simulink model "TrajectoryFollowVehicleWith14DoF"  (R2024a)
settings: Solver=VariableStepAuto  StartTime=0  StopTime=14  FixedStep=timeStep  RelTol=1e-3
PreLoadFcn:
  | useDynamicsStanley = false; %Simulink model to move according to the scenario trajectory.
  | vehicleVariant = "3DOF";
PostLoadFcn:
  | load(fullfile(matlabroot,'toolbox','driving','drivingdata','rrScenarioSimTypes.mat'));
  | helperSLTrajectoryFollowerWithRRScenarioSetup();
  | heightMap = "flat";
  | if isfile("pathFollowingUtil/gridMap_groundHeight_RT.mat")
  |     load("gridMap_groundHeight_RT.mat");
  | end
  | % if exist("z_2DTable", "var") && exist("xBreakPts", "var") && exist("yBreakPts", "var")
  | %     hegihtMap = "2DMap";
  | % end
  | % if isfile("CRG/crgRoad.crg")
  | %     crgData = crg_read('CRG/crgRoad.crg');
  | % end
InitFcn:
  | if ~exist("useLongitudinalEV", "var")
  |     useLongitudinalEV = false;
  | end
StartFcn:
  | % set_param(bdroot, 'Profile', 'on');
StopFcn:
  | % set_param(bdroot, 'Profile', 'off');
  | % slprofreport(bdroot, 'report14DoF.html');
undefined symbols (not defined in the file or in its folder): ActorRuntime, Camera, control_timeStep, Defined, DiscIntNeverNeededParam, dz, Ego, egoInitialPose, egoInitialPoseCG, egoInitialPoseRear, InitVehicle, kmph2mps, Lane, lr, m, magnitude, max_dc, n, numReferencePose, pitch, roll, RRtimeStep, SceneData, SRE, steerGear, tau, tau2, timeStep, User, VehicleData, WheelPoses, X, xBreakPts, Y, yaw, yBreakPts, Z, z_2DTable
libraries: sm_lib x108, nesl_utility x62, sm_vehicle_utilities_lib x30, simulink_extras x12, roadrunnerscenario x6, simulink x4, drivingvehiclecontroller x4, autolibshared x2, mpcadaslib x2, autolibutils x1, METI_Lib_vehicle_model x1
(part 2 of 6)

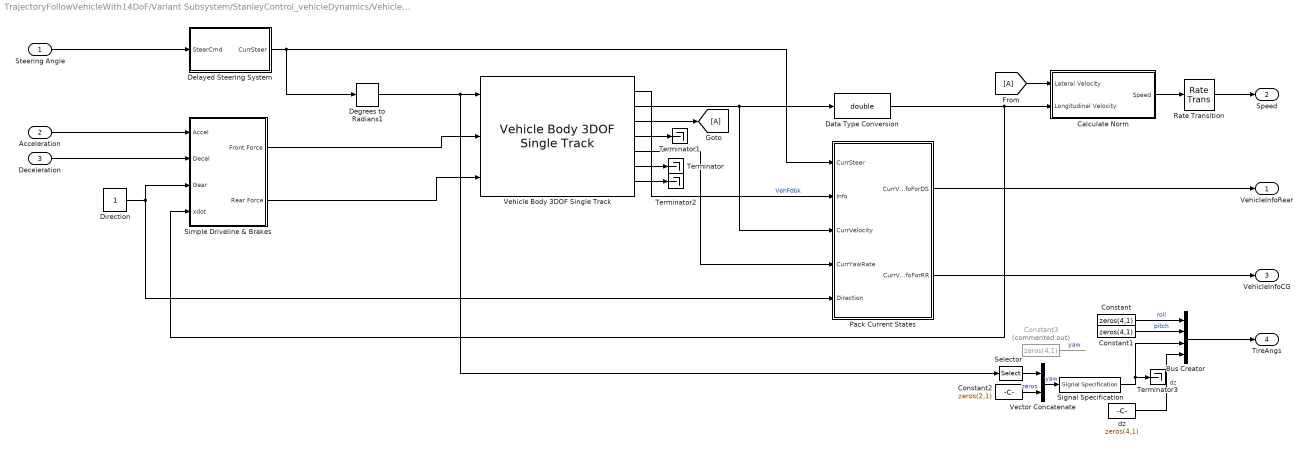
== system TrajectoryFollowVehicleWith14DoF/Variant Subsystem/StanleyControl_vehicleDynamics/Vehicle Dynamics1/Vehicle Dynamics 3DOF ==
  Steering Angle : Inport
  Acceleration : Inport  Port=2
  Deceleration : Inport  Port=3
  Bus Creator : BusCreator  Inputs=roll,pitch,yaw,dz
  Calculate Norm : Subsystem
  Constant : Constant  Value=zeros(4,1)
  Constant1 : Constant  Value=zeros(4,1)
  Constant2 : Constant  Value=zeros(2,1)
  Constant3 : Constant  Commented=on  Value=zeros(4,1)
  Data Type Conversion : DataTypeConversion  OutDataTypeStr=double  SaturateOnIntegerOverflow=off  RndMeth=Floor
  Degrees to Radians1 : simulink_extras/Transformations/Degrees to Radians
  Delayed Steering System : Subsystem
  Direction : Constant
  From : From
  Goto : Goto
  Pack Current States : Subsystem
  Rate Transition : RateTransition
  Selector : Selector  InputPortWidth=1  IndexOptions=Index vector (dialog)  Indices=[1; 1]  OutputSizes=1
  Signal Specification : SignalSpecification  Unit=rad  Dimensions=[4,1]
  Simple Driveline & Brakes : Subsystem
  Terminator{,1..3} (4 alike) : Terminator
  Vector Concatenate : Concatenate  Mode=Multidimensional array
  Vehicle Body 3DOF Single Track : autolibshared/Vehicle Body 3DOF Single Track  trackMode=Single (bicycle)  inputMode=External longitudinal forces  frontSteerMode=on  rearSteerMode=off  windMode=off  muMode=off  extFMode=off  extMMode=off  htchFMode=off  htchMMode=off  extXo=off  extpsio=off  extxdoto=off  extro=off  extYo=off  extTamb=off  extydoto=off  aMode=2  NF=2  NR=2  m=m  a=lf  b=lr  h=0.35  dh=1  hh=0.2  X_o=egoInitialPoseCG.CurrPose(1)  xdot_o=egoInitialPoseCG.CurrVelocity  CalphaMode=off  sigmaMode=off  d=0  hl=0  w=[1.4,1.4]  Cy_f=Cf  Cy_r=Cr  sigma_f=.1  sigma_r=.1  alpha_f_brk=[-.1 .1]  Cy_f_data=[-9e3 9e3]  alpha_r_brk=[-.1 .1]  Cy_r_data=[-9e3 9e3]  Y_o=egoInitialPoseCG.CurrPose(2)  ydot_o=0  Izz=Iz  psi_o=deg2rad(egoInitialPoseCG.CurrPose(3))  r_o=deg2rad(egoInitialPoseCG.CurrYawRate)  Af=0  Cd=.3  Cl=.1  Cpm=.1  beta_w=[0:0.01:0.3]  Cs=[0:0.03:0.9]  Cym=[0:0.01:0.3]  Pabs=101325  Tair=273  g=9.81  mu=1  xdot_tol=.01  Fznom=5000  Fxtire_sat=7e4  Fytire_sat=7e4  longOff=0  latOff=0  vertOff=0  wrapAng=off
  dz : Constant  Value=zeros(4,1)
  VehicleInfoRear : Outport
  Speed : Outport  Port=2
  VehicleInfoCG : Outport  Port=3
  TireAngs : Outport  Port=4
  wires:
  Steering Angle/1 -> Delayed Steering System/1(SteerCmd)
  Acceleration/1 -> Simple Driveline & Brakes/1(Accel)
  Calculate Norm/1(Speed) -> Rate Transition/1
  Direction/1 -> Pack Current States/5(Direction), Simple Driveline & Brakes/3(Gear)
  Simple Driveline & Brakes/1(Front Force) -> Vehicle Body 3DOF Single Track/2
  Vehicle Body 3DOF Single Track/5 -> Pack Current States/4(CurrYawRate)
  Vehicle Body 3DOF Single Track/4 -> Terminator1/1
  Degrees to Radians1/1 -> Selector/1, Vehicle Body 3DOF Single Track/1
  Delayed Steering System/1(CurrSteer) -> Degrees to Radians1/1, Pack Current States/1(CurrSteer)
  Pack Current States/1(CurrVehicleInfoForDS) -> VehicleInfoRear/1
  Rate Transition/1 -> Speed/1
  Simple Driveline & Brakes/2(Rear Force) -> Vehicle Body 3DOF Single Track/3
  From/1 -> Calculate Norm/1(Lateral Velocity)
  Vehicle Body 3DOF Single Track/2 -> Data Type Conversion/1, Pack Current States/3(CurrVelocity)
  Vehicle Body 3DOF Single Track/6 -> Terminator/1
  Deceleration/1 -> Simple Driveline & Brakes/2(Decel)
  Vehicle Body 3DOF Single Track/7 -> Terminator2/1
  Vehicle Body 3DOF Single Track/3 -> Goto/1
  Data Type Conversion/1 -> Calculate Norm/2(Longitudinal Velocity), Simple Driveline & Brakes/4(xdot)
  Vehicle Body 3DOF Single Track/1 -> Pack Current States/2(Info)  "VehFdbk"
  Pack Current States/2(CurrVehicleInfoForRR) -> VehicleInfoCG/1
  Constant/1 -> Bus Creator/1  "roll"
  Constant1/1 -> Bus Creator/2  "pitch"
  Bus Creator/1 -> TireAngs/1
  Vector Concatenate/1 -> Signal Specification/1  "yaw"
  Constant2/1 -> Vector Concatenate/2  "zeros"
  dz/1 -> Bus Creator/4  "dz"
  Constant3/1 -> ?  "yaw"
  Selector/1 -> Vector Concatenate/1
  Signal Specification/1 -> Bus Creator/3, Terminator3/1

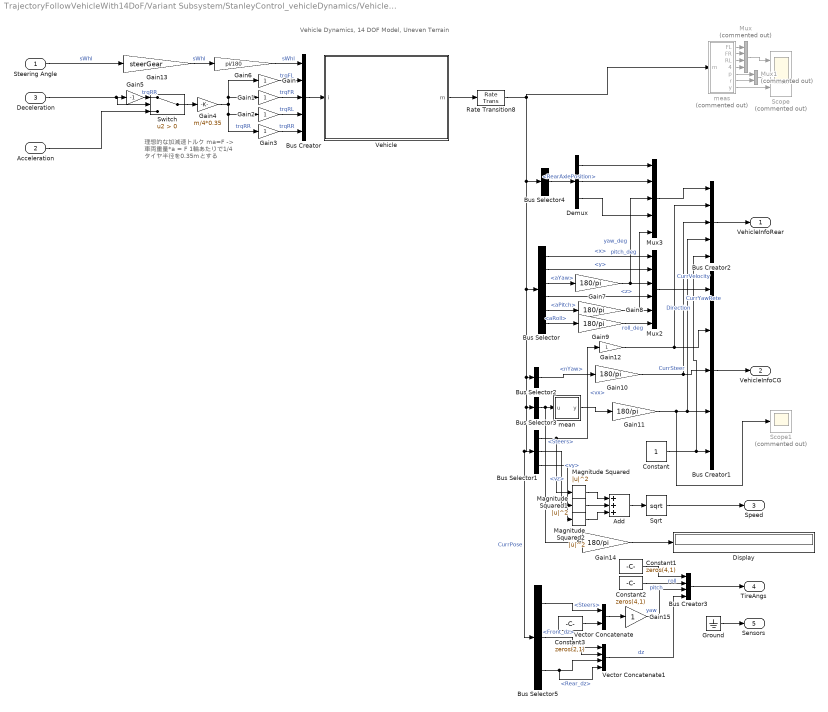
== system TrajectoryFollowVehicleWith14DoF/Variant Subsystem/StanleyControl_vehicleDynamics/Vehicle Dynamics1/Vehicle Dynamics Multibody ==
  note: 理想的な加減速トルク
      | ma=F -> 車両重量*a = F
      | 1輪あたりで1/4
      | タイヤ半径を0.35mとする
  note: Vehicle Dynamics, 14 DOF Model, Uneven Terrain
  Steering Angle : Inport
  Acceleration : Inport  Port=2
  Deceleration : Inport  Port=3
  Add : Sum  Inputs=+++
  Bus Creator : BusCreator  Inputs=5
  Bus Creator1 : BusCreator  Inputs=5  OutDataTypeStr=Bus: BusFullVehicleInfo  NonVirtualBus=on
      settings: InheritFromInputs=off
  Bus Creator2 : BusCreator  Inputs=5  OutDataTypeStr=Bus: BusVehicleInfo  NonVirtualBus=on
      settings: InheritFromInputs=off
  Bus Creator3 : BusCreator  Inputs=4
  Bus Selector : BusSelector  OutputSignals=Body.x,Body.y,Body.aYaw,Body.z,Body.aPitch,Body.aRoll
  Bus Selector1 : BusSelector  OutputSignals=Body.vx,Body.vy,Body.vz
  Bus Selector2 : BusSelector  OutputSignals=Body.nYaw
  Bus Selector3 : BusSelector  OutputSignals=Steers
  Bus Selector4 : BusSelector  OutputSignals=RearAxlePosition
  Bus Selector5 : BusSelector  OutputSignals=Steers,Front_dz,Rear_dz
  Constant : Constant
  Constant1 : Constant  Value=zeros(4,1)
  Constant2 : Constant  Value=zeros(4,1)
  Constant3 : Constant  Value=zeros(2,1)
  Demux : Demux  Outputs=3
  Display : Display
  Gain{,1..3,12,15} (6 alike) : Gain
  Gain{7..11,14} (6 alike) : Gain  Gain=180/pi
  Gain13 : Gain  Gain=steerGear
  Gain4 : Gain  Gain=m/4*0.35
  Gain5 : Gain  Gain=-1
  Gain6 : Gain  Gain=pi/180
  Ground : Ground
  Magnitude Squared : Math  Operator=magnitude^2
  Magnitude Squared1 : Math  Operator=magnitude^2
  Magnitude Squared2 : Math  Operator=magnitude^2
  Mux : Mux  Commented=on
  Mux1 : Mux  Commented=on  Inputs=2
  Mux2 : Mux  Inputs=6
  Mux3 : Mux  Inputs=5
  Rate Transition8 : RateTransition  OutPortSampleTime=timeStep
  Scope : Scope  Commented=on  NumInputPorts=3
  Scope1 : Scope  Commented=on
  Sqrt : Sqrt  OutputSignalType=real
  Switch : Switch  Criteria=u2 > Threshold  SaturateOnIntegerOverflow=off  InputSameDT=off
  Vector Concatenate : Concatenate
  Vector Concatenate1 : Concatenate  NumInputs=4
  Vehicle : Subsystem  mask(Vehicle and Scene){vehdata=VehicleData, initveh=InitVehicle}
      mask prompts: vehdata "Vehicle Data (structure)"; initveh "Initial Position, Velocity (structure)"
      mask help: Models a vehicle with a configurable scene. Vehicle parameters are defined within a single data structure. A separate data structure defines the initial position, orientation, and speed of the vehicle and the wheels.
      settings: AttributesFormatString=%<popup_scene>
      mask Display:
      | image(['sm_vehicle_2axle_heave_roll_vehicle_grid_ray_trace.png']);
      | % Notes for mask images
      | % Screenshot taken MechExp 931x463, one pane 619x314
      | % Trim to 434 x 272, resize to 500x330
  mean : MATLAB Function  TreatAsAtomicUnit=on
  meas : Subsystem  Commented=on
  VehicleInfoRear : Outport
  VehicleInfoCG : Outport  Port=2
  Speed : Outport  Port=3
  TireAngs : Outport  Port=4
  Sensors : Outport  Port=5
  wires:
  Demux/3 -> Mux3/4
  Magnitude Squared2/1 -> Add/3
  Gain11/1 -> Scope1/1, Bus Creator1/4, Bus Creator2/4  "CurrSteer"
  Demux/1 -> Mux3/1
  Bus Creator1/1 -> VehicleInfoCG/1
  Bus Selector1/1 -> Gain12/1, Magnitude Squared/1  "<vx>"
  Bus Creator2/1 -> VehicleInfoRear/1
  Mux2/1 -> Bus Creator1/1
  Bus Selector/4 -> Mux2/4  "<z>"
  Gain13/1 -> Gain6/1  "sWhl"
  Gain6/1 -> Bus Creator/1  "sWhl"
  Sqrt/1 -> Speed/1
  Bus Selector1/2 -> Magnitude Squared1/1  "<vy>"
  Bus Selector3/1 -> Gain14/1, mean/1(u)  "<Steers>"
  Bus Selector/5 -> Gain8/1  "<aPitch>"
  Gain12/1 -> Bus Creator1/2, Bus Creator2/2  "CurrVelocity"
  Bus Selector2/1 -> Gain10/1  "<nYaw>"
  Gain10/1 -> Bus Creator2/3, Bus Creator1/3  "CurrYawRete"
  Bus Selector/1 -> Mux2/1  "<x>"
  Constant/1 -> Bus Creator2/5, Bus Creator1/5  "Direction"
  Mux3/1 -> Bus Creator2/1
  Bus Selector/2 -> Mux2/2  "<y>"
  Magnitude Squared/1 -> Add/1
  Magnitude Squared1/1 -> Add/2
  Gain7/1 -> Mux3/3, Mux2/3  "yaw_deg"
  Acceleration/1 -> Switch/3
  Mux/1 -> Scope/1
  meas/3(RL) -> Mux/3
  Demux/2 -> Mux3/2
  Bus Selector1/3 -> Magnitude Squared2/1  "<vz>"
  Vehicle/1(m) -> Rate Transition8/1
  Gain3/1 -> Bus Creator/5  "trqRR"
  Bus Selector/3 -> Gain7/1  "<aYaw>"
  Switch/1 -> Gain4/1
  Gain4/1 -> Gain1/1, Gain/1, Gain2/1, Gain3/1  "trqRR"
  Add/1 -> Sqrt/1
  Gain5/1 -> Switch/1  "trqRR"
  Gain/1 -> Bus Creator/2  "trqFL"
  mean/1(y) -> Gain11/1
  Bus Creator/1 -> Vehicle/1(i)
  meas/2(FR) -> Mux/2
  meas/1(FL) -> Mux/1
  Gain1/1 -> Bus Creator/3  "trqFR"
  Gain9/1 -> Mux2/6  "roll_deg"
  meas/6(r) -> Mux1/2
  meas/7(y) -> Scope/3
  Steering Angle/1 -> Gain13/1  "sWhl"
  Deceleration/1 -> Switch/2, Gain5/1
  Mux1/1 -> Scope/2
  meas/4(RR) -> Mux/4
  Gain8/1 -> Mux3/5, Mux2/5  "pitch_deg"
  Bus Selector4/1 -> Demux/1  "<RearAxlePosition>"
  Gain2/1 -> Bus Creator/4  "trqRL"
  Bus Selector/6 -> Gain9/1  "<aRoll>"
  meas/5(p) -> Mux1/1
  Rate Transition8/1 -> meas/1(m), Bus Selector5/1, Bus Selector1/1, Bus Selector3/1, Bus Selector2/1, Bus Selector/1, Bus Selector4/1  "CurrPose"
  Gain14/1 -> Display/1
  Vector Concatenate/1 -> Gain15/1
  Constant1/1 -> Bus Creator3/1  "roll"
  Constant2/1 -> Bus Creator3/2  "pitch"
  Gain15/1 -> Bus Creator3/3  "yaw"
  Bus Creator3/1 -> TireAngs/1
  Vector Concatenate1/1 -> Bus Creator3/4  "dz"
  Ground/1 -> Sensors/1
  Constant3/1 -> Vector Concatenate/2
  Bus Selector5/1 -> Vector Concatenate/1  "<Steers>"
  Bus Selector5/2 -> Vector Concatenate1/2, Vector Concatenate1/1  "<Front_dz>"
  Bus Selector5/3 -> Vector Concatenate1/4, Vector Concatenate1/3  "<Rear_dz>"

== system TrajectoryFollowVehicleWith14DoF/Variant Subsystem/LongitudinalEV/VDBS_PTBS/Controllers/Powertrain Control Input ==
  OpCmds : Inport
  VehPlnt : Inport  Port=2
  Bus Selector1 : BusSelector  OutputSignals=Veh.xdot,Veh.MotSpd,Elec.BMS_Sensors
  Bus Selector2 : BusSelector  OutputSignals=Accel,Decel
  Rate Transition{,1..2,6} (4 alike) : RateTransition  Deterministic=off
  AccelPdl : Outport  VectorParamsAs1DForOutWhenUnconnected=off
  DecelPdl : Outport  Port=2  VectorParamsAs1DForOutWhenUnconnected=off
  VehSpdFdbk : Outport  Port=3  VectorParamsAs1DForOutWhenUnconnected=off
  MotSpd : Outport  Port=4  VectorParamsAs1DForOutWhenUnconnected=off
  BMS_Sensors : Outport  Port=5  OutDataTypeStr=Bus: Sensors  VectorParamsAs1DForOutWhenUnconnected=off
  wires:
  OpCmds/1 -> Bus Selector2/1
  VehPlnt/1 -> Bus Selector1/1
  Bus Selector2/1 -> Rate Transition/1  "<Accel>"
  Bus Selector2/2 -> Rate Transition1/1  "<Decel>"
  Bus Selector1/1 -> Rate Transition2/1  "<xdot>"
  Bus Selector1/2 -> Rate Transition6/1  "<MotSpd>"
  Rate Transition/1 -> AccelPdl/1
  Rate Transition1/1 -> DecelPdl/1
  Rate Transition2/1 -> VehSpdFdbk/1
  Rate Transition6/1 -> MotSpd/1
  Bus Selector1/3 -> BMS_Sensors/1  "<BMS_Sensors>"

== system TrajectoryFollowVehicleWith14DoF/Variant Subsystem/LongitudinalEV/VDBS_PTBS/Controllers/Powertrain Control Module (PCM) ==
  AccCmd : Inport
  DecCmd : Inport  Port=2
  VehSpdFdbk : Inport  Port=3
  MotSpd : Inport  Port=4
  BMS_Sensors : Inport  Port=5  OutDataTypeStr=Bus: Sensors
  Battery Management System (BMS) : ModelReference  ModelNameDialog=BMS_Software.slx  ModelReferenceVersion=8.0
  Enumerated Constant : simulink/Sources/Enumerated Constant  OutDataTypeStr=Enum: SRE  Value=SRE.Driving  SampleTime=inf
  Powertrain Control Module (PCM) : ModelReference  ModelNameDialog=EvPowertrainController.slx  ModelReferenceVersion=8.4
  MotTrqCmd : Outport
  BrakeCmd : Outport  Port=2
  BMS_Info : Outport  Port=3  OutDataTypeStr=Bus: BMS_Info
  BMS_Cmd : Outport  Port=4  OutDataTypeStr=Bus: BMS_Cmd
  wires:
  DecCmd/1 -> Powertrain Control Module (PCM)/2
  Powertrain Control Module (PCM)/1 -> MotTrqCmd/1
  [BMS_Info] -> Powertrain Control Module (PCM)/4
  MotSpd/1 -> Powertrain Control Module (PCM)/6
  VehSpdFdbk/1 -> Powertrain Control Module (PCM)/3
  AccCmd/1 -> Powertrain Control Module (PCM)/1
  Powertrain Control Module (PCM)/2 -> BrakeCmd/1
  Enumerated Constant/1 -> Battery Management System (BMS)/1
  Battery Management System (BMS)/1 -> [BMS_Info], BMS_Info/1
  Battery Management System (BMS)/2 -> [BMS_Cmd], BMS_Cmd/1
  BMS_Sensors/1 -> Powertrain Control Module (PCM)/7, Battery Management System (BMS)/2
  [BMS_Cmd] -> Powertrain Control Module (PCM)/5

== system TrajectoryFollowVehicleWith14DoF/Variant Subsystem/LongitudinalEV/VDBS_PTBS/Controllers/Powertrain Control Output ==
  MotTrqCmd : Inport
  BrkCmd : Inport  Port=2
  BMS_Info : Inport  Port=3  OutDataTypeStr=Bus: BMS_Info
  BMS_Cmd : Inport  Port=4  OutDataTypeStr=Bus: BMS_Cmd
  Bus Creator : BusCreator  Inputs=4
  PtCtrl : Outport  VectorParamsAs1DForOutWhenUnconnected=off
  wires:
  BrkCmd/1 -> Bus Creator/2  "BrkCmd"
  Bus Creator/1 -> PtCtrl/1  "PtCtrl"
  MotTrqCmd/1 -> Bus Creator/1  "MotTrqCmd"
  BMS_Info/1 -> Bus Creator/3  "BMS_Info"
  BMS_Cmd/1 -> Bus Creator/4  "BMS_Cmd"

== system TrajectoryFollowVehicleWith14DoF/Variant Subsystem/LongitudinalEV/VDBS_PTBS/Longitudinal Driver/Longitudinal Driver ==
  Vref : Inport
  Vfdbk : Inport  Port=2
  Bus Selector : BusSelector  OutputSignals=Veh.xdot
  Ground : Ground
  Longitudinal Driver Model : autolibshared/Longitudinal Driver  extAccelOvr=off  extDecelOvr=off  extAccelHld=off  extDecelHld=off  extAccelZero=off  extDecelZero=off  cntrlType=Predictive  shftType=Reverse, Neutral, Drive  velUnits=m/s  gearOut=off  Kp=1  Ki=1  Kff=0  Kg=0  VehVelVec=[0 100]  KffVec=[.1 .1]  KpVec=[10 10]  KiVec=[5 5]  KgVec=[0 0]  m=1645  Kpt=450*9.04/0.324  tau=0.12  L=4  aR=30.3/3875  bR=0.21290*4.44822/0.44704  cR=0.01278*4.44822/0.44704^2  g=9.81  vnom=1  Kaw=0  tauerr=0  tauPt=2  GearInit=0  tShift=.1  pdlVec=[0.1 0.4 0.5 0.9]  upShftTbl=[-1 12.9375 26.4375 39.9375 51.18749999999999 62.4375 72.84375 83.25;-1 16.3125 29.8125 43.3125 54.5624 65.8125 76.78125 87.75;-1 19.6875 33.1875 46.68749999999999 57.9375 69.1875 80.71875 92.25;-1 33 52.5 77.25 100.5 138.75 161.875 185]  dwnShftTbl=[1 9.5625 23.0625 36.5625 47.8125 59.0625 68.90625 78.75;1 12.9375 26.4375 39.9375 51.18749999999999 62.4375 72.84375 83.25;1 16.3125 29.8125 43.3125 54.562499 65.8125 76.78125 87.75;1 19.6875 33.1875 46.68749999999999 57.9375 69.1875 80.71875 92.25]  tClutch=.5  tRev=.5  tPark=120  aMode=1  UpGearVec="[0  1  2  3  4  5  6  7]"  DownGearVec="[1  2  3  4  5  6  7  8]"
  Terminator1 : Terminator
  OpCmds : Outport  VectorParamsAs1DForOutWhenUnconnected=off
  tag scope: Accel_VDBS=global
  wires:
  Bus Selector/1 -> Longitudinal Driver Model/2  "<xdot>"
  Vref/1 -> Longitudinal Driver Model/1  "xdotref"
  Vfdbk/1 -> Bus Selector/1
  Longitudinal Driver Model/2 -> [Accel_VDBS]  "Acc"
  Longitudinal Driver Model/3 -> Terminator1/1  "Dec"
  Ground/1 -> Longitudinal Driver Model/3
  Longitudinal Driver Model/1 -> OpCmds/1  "Info"

== system TrajectoryFollowVehicleWith14DoF/Variant Subsystem/LongitudinalEV/VDBS_PTBS/Longitudinal Driver/Open Loop ==
  note: This subsystem is provided to disable the driver subsystem and expose the driver interface.
      |
      | The interface can:
      | - be connected with dashboard UI blocks or 3rd party hardware
      | - provide application specific pre-programmed event or time based signals
      | - be driven by recorded operator signals for tuning, troubleshooting and model validation
  Bus Creator2 : BusCreator  Inputs=8
  Constant{1..4} (4 alike) : Constant  Value=0
  Ground{,1..3} (4 alike) : Ground
  OpCmds : Outport  VectorParamsAs1DForOutWhenUnconnected=off
  wires:
  Ground3/1 -> Bus Creator2/8  "ErrMin"
  Ground1/1 -> Bus Creator2/6  "ErrSqrSum"
  Bus Creator2/1 -> OpCmds/1  "Info"
  Ground2/1 -> Bus Creator2/7  "ErrMax"
  Constant1/1 -> Bus Creator2/1  "Accel"
  Constant3/1 -> Bus Creator2/3  "Gear"
  Constant2/1 -> Bus Creator2/2  "Decel"
  Ground/1 -> Bus Creator2/5  "Err"
  Constant4/1 -> Bus Creator2/4  "Clutch"

== system TrajectoryFollowVehicleWith14DoF/Variant Subsystem/LongitudinalEV/VDBS_PTBS/Passenger Car/Drivetrain Output ==
  VehSpd : Inport
  MotSpd : Inport  Port=2
  Bus Creator1 : BusCreator  Inputs=2
  VehFdbk : Outport  VectorParamsAs1DForOutWhenUnconnected=off
  wires:
  Bus Creator1/1 -> VehFdbk/1  "VehFdbk"
  VehSpd/1 -> Bus Creator1/1
  MotSpd/1 -> Bus Creator1/2  "MotSpd"

== system TrajectoryFollowVehicleWith14DoF/Variant Subsystem/LongitudinalEV/VDBS_PTBS/Passenger Car/Drivetrain Plant Input ==
  Ctrl : Inport
  ElecFdbk : Inport  Port=2
  Env : Inport  Port=3
  Bus Selector : BusSelector  OutputSignals=BrkCmd
  Bus Selector1 : BusSelector  OutputSignals=MotTrq
  Bus Selector3 : BusSelector  OutputSignals=Ground.Grade,Wind.wind_x
  First Order Hold : FirstOrderHold  ErrorTolerance=inf
  Rate Transition6 : RateTransition  Deterministic=off
  Rate Transition7 : RateTransition  Deterministic=off
  MotTrq : Outport  VectorParamsAs1DForOutWhenUnconnected=off
  BrkCmd : Outport  Port=2  VectorParamsAs1DForOutWhenUnconnected=off
  Grade : Outport  Port=3  VectorParamsAs1DForOutWhenUnconnected=off
  WindVel : Outport  Port=4  VectorParamsAs1DForOutWhenUnconnected=off
  wires:
  Ctrl/1 -> Bus Selector/1
  Bus Selector/1 -> First Order Hold/1  "<BrkCmd>"
  First Order Hold/1 -> BrkCmd/1  "BrkCmd"
  ElecFdbk/1 -> Bus Selector1/1
  Bus Selector1/1 -> MotTrq/1  "<MotTrq>"
  Env/1 -> Bus Selector3/1
  Rate Transition6/1 -> Grade/1  "Grade"
  Rate Transition7/1 -> WindVel/1  "WindVel"
  Bus Selector3/1 -> Rate Transition6/1  "<Grade>"
  Bus Selector3/2 -> Rate Transition7/1  "<wind_x>"

== system TrajectoryFollowVehicleWith14DoF/Variant Subsystem/LongitudinalEV/VDBS_PTBS/Passenger Car/Electric Plant ==
  MotTrqCmd : Inport
  MotSpd : Inport  Port=2
  AmbTmp : Inport  Port=3
  BMS_Info : Inport  Port=4  OutDataTypeStr=Bus: BMS_Info
  BMS_Cmd : Inport  Port=5  OutDataTypeStr=Bus: BMS_Cmd
  VehSpd : Inport  Port=6
  Powertrain Blockset : Subsystem  VariantControl=Powertrain Blockset
  Simscape : ModelReference  ModelNameDialog=BattEv_Simscape.slx  VariantControl=Simscape  ModelReferenceVersion=5.0
  BattSoc : Outport
  BattPwr : Outport  Port=2
  BattCrnt : Outport  Port=3
  MotTrq : Outport  Port=4
  BMS_Sensors : Outport  Port=5  OutDataTypeStr=Bus: Sensors

== system TrajectoryFollowVehicleWith14DoF/Variant Subsystem/LongitudinalEV/VDBS_PTBS/Passenger Car/Electric Plant Input ==
  Ctrl : Inport
  Veh : Inport  Port=2
  Env : Inport  Port=3
  Bus Selector : BusSelector  OutputSignals=MotTrqCmd,BMS_Info,BMS_Cmd
  Bus Selector1 : BusSelector  OutputSignals=MotSpd,xdot
  Bus Selector2 : BusSelector  OutputSignals=Temp
  First Order Hold : FirstOrderHold  ErrorTolerance=inf
  MotTrqCmd : Outport  VectorParamsAs1DForOutWhenUnconnected=off
  MotSpd : Outport  Port=2  VectorParamsAs1DForOutWhenUnconnected=off
  AmbTmp : Outport  Port=3  VectorParamsAs1DForOutWhenUnconnected=off
  BMS_Info : Outport  Port=4  OutDataTypeStr=Bus: BMS_Info  VectorParamsAs1DForOutWhenUnconnected=off
  BMS_Cmd : Outport  Port=5  OutDataTypeStr=Bus: BMS_Cmd  VectorParamsAs1DForOutWhenUnconnected=off
  VehSpd : Outport  Port=6  VectorParamsAs1DForOutWhenUnconnected=off
  wires:
  First Order Hold/1 -> MotTrqCmd/1  "MotTrqCmd"
  Ctrl/1 -> Bus Selector/1
  Bus Selector/1 -> First Order Hold/1  "<MotTrqCmd>"
  Veh/1 -> Bus Selector1/1
  Bus Selector1/1 -> MotSpd/1  "<MotSpd>"
  Env/1 -> Bus Selector2/1
  Bus Selector2/1 -> AmbTmp/1  "<Temp>"
  Bus Selector/2 -> BMS_Info/1  "<BMS_Info>"
  Bus Selector/3 -> BMS_Cmd/1  "<BMS_Cmd>"
  Bus Selector1/2 -> VehSpd/1  "<xdot>"

== system TrajectoryFollowVehicleWith14DoF/Variant Subsystem/LongitudinalEV/VDBS_PTBS/Passenger Car/Electric Plant Output ==
  BattSoc : Inport
  BattPwr : Inport  Port=2
  BattCrnt : Inport  Port=3
  MotTrq : Inport  Port=4
  BMS_Sensors : Inport  Port=5  OutDataTypeStr=Bus: Sensors
  Bus Creator1 : BusCreator  Inputs=5
  ElecFdbk : Outport  VectorParamsAs1DForOutWhenUnconnected=off
  wires:
  Bus Creator1/1 -> ElecFdbk/1  "ElecFdbk"
  BattPwr/1 -> Bus Creator1/2
  BattCrnt/1 -> Bus Creator1/3
  MotTrq/1 -> Bus Creator1/4
  BMS_Sensors/1 -> Bus Creator1/5
  BattSoc/1 -> Bus Creator1/1

== system TrajectoryFollowVehicleWith14DoF/Variant Subsystem/LongitudinalEV/VDBS_PTBS/Visualization/Performance Calculations ==
  BattPwr : Inport
  VehSpd : Inport  Port=2
  Divide : Product  Inputs=*/
  Divide1 : Product  Inputs=*/
  Divide2 : Product  Inputs=*/
  Integrator : Integrator
  Integrator1 : Integrator
  L/100 Km Calc : Product  Inputs=/*
  Product : Product
  Saturation : Saturate  UpperLimit=Inf  LowerLimit=0.001  ZeroCross=off
  Saturation1 : Saturate  UpperLimit=Inf  LowerLimit=1e-3  ZeroCross=off
  Sqrt : Sqrt
  US EPA kwh/USgal equivalent : Constant  Value=33.7
  US MPG Calc : Product  Inputs=*/
  m to 100Km : Gain  Gain=1/1000/100
  m to mile : Gain  Gain=0.000621371
  m^3 per gal : Gain  Gain=0.00378541
  m^3 to L : Gain  Gain=1000
  m^3 to US Gal : Gain  Gain=264.172
  s per h : Constant  Value=3600
  w per kw : Constant  Value=1000
  US MPG : Outport  VectorParamsAs1DForOutWhenUnconnected=off
  L/100Km : Outport  Port=2  VectorParamsAs1DForOutWhenUnconnected=off
  wires:
  m^3 to US Gal/1 -> Saturation1/1
  m^3 to L/1 -> L/100 Km Calc/2
  Integrator/1 -> m to mile/1, m to 100Km/1
  m to mile/1 -> US MPG Calc/1
  Integrator1/1 -> m^3 to US Gal/1, m^3 to L/1
  Saturation/1 -> L/100 Km Calc/1
  m to 100Km/1 -> Saturation/1
  L/100 Km Calc/1 -> L/100Km/1  "L/100Km"
  Saturation1/1 -> US MPG Calc/2
  US MPG Calc/1 -> US MPG/1  "US MPG"
  w per kw/1 -> Divide/2
  Divide/1 -> Divide2/1
  Divide2/1 -> Divide1/1
  s per h/1 -> Divide1/2
  Divide1/1 -> m^3 per gal/1
  m^3 per gal/1 -> Integrator1/1
  US EPA kwh/USgal equivalent/1 -> Divide2/2
  BattPwr/1 -> Divide/1
  Sqrt/1 -> Integrator/1
  Product/1 -> Sqrt/1
  VehSpd/1 -> Product/2, Product/1

== system TrajectoryFollowVehicleWith14DoF/Variant Subsystem/LongitudinalEV/VDBS_PTBS/Visualization/Performance Calculations instant ==
  BattPwr : Inport
  VehSpd : Inport  Port=2
  Divide : Product  Inputs=*/
  Divide1 : Product  Inputs=*/
  Divide2 : Product  Inputs=*/
  L/100 Km Calc : Product  Inputs=/*
  Product : Product
  Saturation : Saturate  UpperLimit=Inf  LowerLimit=0.001  ZeroCross=off
  Saturation1 : Saturate  UpperLimit=Inf  LowerLimit=1e-3  ZeroCross=off
  Sqrt : Sqrt
  US EPA kwh/USgal equivalent : Constant  Value=33.7
  US MPG Calc : Product  Inputs=*/
  m to 100Km : Gain  Gain=1/1000/100
  m to mile : Gain  Gain=0.000621371
  m^3 per gal : Gain  Gain=0.00378541
  m^3 to L : Gain  Gain=1000
  m^3 to US Gal : Gain  Gain=264.172
  s per h : Constant  Value=3600
  w per kw : Constant  Value=1000
  US MPG : Outport  VectorParamsAs1DForOutWhenUnconnected=off
  L/100Km : Outport  Port=2  VectorParamsAs1DForOutWhenUnconnected=off
  wires:
  VehSpd/1 -> Product/1, Product/2
  Product/1 -> Sqrt/1
  BattPwr/1 -> Divide/1
  US EPA kwh/USgal equivalent/1 -> Divide2/2
  Divide1/1 -> m^3 per gal/1
  s per h/1 -> Divide1/2
  Divide2/1 -> Divide1/1
  Divide/1 -> Divide2/1
  w per kw/1 -> Divide/2
  US MPG Calc/1 -> US MPG/1  "US MPG"
  Saturation1/1 -> US MPG Calc/2
  L/100 Km Calc/1 -> L/100Km/1  "L/100Km"
  m to 100Km/1 -> Saturation/1
  Saturation/1 -> L/100 Km Calc/1
  m^3 per gal/1 -> m^3 to L/1, m^3 to US Gal/1
  m to mile/1 -> US MPG Calc/1
  Sqrt/1 -> m to 100Km/1, m to mile/1
  m^3 to L/1 -> L/100 Km Calc/2
  m^3 to US Gal/1 -> Saturation1/1

== system TrajectoryFollowVehicleWith14DoF/Variant Subsystem/LongitudinalEV/VDBS_PTBS/Visualization/電費計算1 ==
  note: km
  note: m
  note: m/s
  note: W
  note: kWh
  note: kWsec
  note: Wsec
  v_vehicle : Inport
  P_Hi_batt : Inport  Port=2
  Constant : Constant  Value=0
  Divide_0wari : METI_Lib_vehicle_model/Divide_0wari
  Gain1 : Gain  Gain=1/1000
  Gain2 : Gain  Gain=1/3600
  Gain7 : Gain  Gain=1/1000
  Integrator : Integrator
  Integrator1 : Integrator
  Saturation Dynamic : simulink/Discontinuities/Saturation Dynamic  OutMin=[]  OutMax=[]  OutDataTypeStr=Inherit: Same as second input  OutDataType=fixdt(1, 16)  OutScaling=2^-10  DoSatur=off
  燃費表示上の上限値 : Constant  Value=50
  Out1 : Outport
  wires:
  Gain7/1 -> Divide_0wari/1
  燃費表示上の上限値/1 -> Saturation Dynamic/1
  Saturation Dynamic/1 -> Out1/1
  Divide_0wari/1 -> Saturation Dynamic/2
  Constant/1 -> Saturation Dynamic/3
  v_vehicle/1 -> Integrator/1
  Integrator/1 -> Gain7/1
  Gain2/1 -> Divide_0wari/2
  P_Hi_batt/1 -> Integrator1/1
  Integrator1/1 -> Gain1/1
  Gain1/1 -> Gain2/1

== system TrajectoryFollowVehicleWith14DoF/Variant Subsystem/StanleyControl_vehicleDynamics/Variant Subsystem/MPC/Path Following wrapper ==
  Set velocity : Inport
  Longitudinal velocity : Inport  Port=2
  Curvature : Inport  Port=3
  Lateral deviation : Inport  Port=4
  Relative yaw angle : Inport  Port=5
  Time gap : Inport  Port=6
  Relative distance : Inport  Port=7
  Relative velocity : Inport  Port=8
  Path Following Control System : mpcadaslib/Path Following Control System  VariantControl=true  ModelType=Use vehicle parameters  VehicleMass=m  VehicleYawInertia=Iz  LengthToFront=lf  LengthToRear=lr  FrontTireStiffness=Cf  RearTireStiffness=Cr  AccelTimeConstant=tau  EgoModelMatrixA=[-2,zeros(1,3);1,zeros(1,3);zeros(1,2),-4.4021,-12.4603;zeros(1,2),1.3913,-5.1868]  EgoModelMatrixB=[2,zeros(1,3);zeros(1,2),24.1270,15.8609]'  EgoModelMatrixC=[zeros(3,1),eye(3)]  InitialLongVel=norm(egoInitialPose.Velocity)  TransportLag=tau2  spaceCtrl=off  DefaultSpacing=0  MinSteering=min_steer  umin_ext=off  MaxSteering=max_steer  umax_ext=off  MinAcceleration=-max_dc  amin_ext=off  MaxAcceleration=max_ac  amax_ext=off  Ts=control_timeStep  PredictionHorizon=PredictionHorizon  ControlHorizon=3  LongWeight=0.1  LateralWeight=1  AccelRateWeight=0.1  SteerRateWeight=0.1  suboptimal=off  maxiter=10  datatypeopt=double  optmode=off  trackmode=off
      settings: LibrarySourceBlock=mpclib/Automated Driving/Path Following Control System
  Longitudinal acceleration : Outport  PortDimensions=1  VectorParamsAs1DForOutWhenUnconnected=off
  Steering angle : Outport  Port=2  VectorParamsAs1DForOutWhenUnconnected=off

== system TrajectoryFollowVehicleWith14DoF/Variant Subsystem/StanleyControl_vehicleDynamics/Vehicle Dynamics1/Vehicle Dynamics 14DOF/3DVisualization ==
  note: 1) Add Subsystem or Model blocks as valid variant choices.
      | 2) You cannot connect blocks at this level. At simulation, connectivity is automatically
      | determined, based on the active variant and port name matching.
  VehFdbk : Inport
  3D Engine : Subsystem  VariantControl=debug_engine3D==true
  No 3D Engine : Subsystem  VariantControl=debug_engine3D==false

== system TrajectoryFollowVehicleWith14DoF/Variant Subsystem/StanleyControl_vehicleDynamics/Vehicle Dynamics1/Vehicle Dynamics 14DOF/Calculate Norm ==
  Longitudinal Velocity : Inport
  Lateral Velocity : Inport  Port=2
  z Velocity : Inport  Port=3
  Add : Sum  Inputs=+++
  Math Function : Math  Operator=square
  Math Function1 : Math  Operator=square
  Math Function2 : Math  Operator=square
  Sqrt : Sqrt
  Speed : Outport
  wires:
  Longitudinal Velocity/1 -> Math Function1/1
  Lateral Velocity/1 -> Math Function/1
  Sqrt/1 -> Speed/1
  Math Function/1 -> Add/1
  Math Function1/1 -> Add/2
  Add/1 -> Sqrt/1
  Math Function2/1 -> Add/3
  z Velocity/1 -> Math Function2/1

== system TrajectoryFollowVehicleWith14DoF/Variant Subsystem/StanleyControl_vehicleDynamics/Vehicle Dynamics1/Vehicle Dynamics 14DOF/Delayed Steering System ==
  SteerCmd : Inport
  Add : Sum  Inputs=+-
  Delay : TransferFcn  Denominator=[0.1 0]
  CurrSteer : Outport  VectorParamsAs1DForOutWhenUnconnected=off
  wires:
  Delay/1 -> Add/2, CurrSteer/1
  SteerCmd/1 -> Add/1
  Add/1 -> Delay/1

== system TrajectoryFollowVehicleWith14DoF/Variant Subsystem/StanleyControl_vehicleDynamics/Vehicle Dynamics1/Vehicle Dynamics 14DOF/Variant Subsystem ==
  note: 1) Add Subsystem or Model blocks as valid variant choices.
      | 2) You cannot connect blocks at this level. At simulation, connectivity is automatically
      | determined, based on the active variant and port name matching.
  VehFdback : Inport
  2DHeightMap : Subsystem  VariantControl="heightMap == \"2DMap\""
  CRG : Subsystem  VariantControl="heightMap == \"CRG\""
  noElevation : Subsystem  VariantControl="heightMap == \"flat\""
  WheelElevation : Outport

== system TrajectoryFollowVehicleWith14DoF/Variant Subsystem/StanleyControl_vehicleDynamics/Vehicle Dynamics1/Vehicle Dynamics 14DOF/getPoseCG ==
  VehFdbk : Inport
  Bus Selector2 : BusSelector  OutputSignals=Body.InertFrm.Cg.Disp.X,Body.InertFrm.Cg.Disp.Y,Body.InertFrm.Cg.Ang.psi,Body.InertFrm.Cg.Disp.Z,Body.InertFrm.Cg.Ang.theta,Body.InertFrm.Cg.Ang.phi
  Gain{4..7} (4 alike) : Gain  Gain=-1
  Math Function2 : Math  Operator=transpose  SignedPower=on
  Mux2 : Mux  Inputs=6
  Radians to Degrees3 : simulink_extras/Transformations/Radians to Degrees
  Radians to Degrees4 : simulink_extras/Transformations/Radians to Degrees
  Radians to Degrees5 : simulink_extras/Transformations/Radians to Degrees
  pitch : Display  Commented=on
  roll : Display  Commented=on
  x : Display  Commented=on
  y : Display  Commented=on
  yaw : Display  Commented=on
  z : Display  Commented=on
  CurrPose : Outport
  wires:
  Bus Selector2/5 -> Radians to Degrees4/1  "<theta>"
  Bus Selector2/6 -> Radians to Degrees5/1  "<phi>"
  Gain4/1 -> y/1, Mux2/2
  Radians to Degrees5/1 -> roll/1, Mux2/6
  Gain5/1 -> z/1, Mux2/4
  Gain7/1 -> pitch/1, Mux2/5
  Bus Selector2/3 -> Radians to Degrees3/1  "<psi>"
  Bus Selector2/2 -> Gain4/1  "<Y>"
  Bus Selector2/1 -> Mux2/1, x/1  "<X>"
  Gain6/1 -> yaw/1, Mux2/3
  Radians to Degrees4/1 -> Gain7/1
  Mux2/1 -> Math Function2/1
  Bus Selector2/4 -> Gain5/1  "<Z>"
  Radians to Degrees3/1 -> Gain6/1
  Math Function2/1 -> CurrPose/1  "CurrPose"
  VehFdbk/1 -> Bus Selector2/1

== system TrajectoryFollowVehicleWith14DoF/Variant Subsystem/StanleyControl_vehicleDynamics/Vehicle Dynamics1/Vehicle Dynamics 14DOF/getPoseRear ==
  VehFdbk : Inport
  Bus Selector1 : BusSelector  OutputSignals=Body.InertFrm.RearAxl.Lft.Disp.X,Body.InertFrm.RearAxl.Rght.Disp.X,Body.InertFrm.RearAxl.Lft.Disp.Y,Body.InertFrm.RearAxl.Rght.Disp.Y,Body.InertFrm.Cg.Ang.psi,Body.InertFrm.RearAxl.Lft.Disp.Z,Body.InertFrm.RearAxl.Rght.Disp.Z,Body.InertFrm.Cg.Ang.theta
  Gain{,1..3} (4 alike) : Gain  Gain=-1
  Math Function1 : Math  Operator=transpose  SignedPower=on
  Mean : Subsystem
  Mean1 : Subsystem
  Mean2 : Subsystem
  Mux1 : Mux  Inputs=5
  Radians to Degrees1 : simulink_extras/Transformations/Radians to Degrees
  Radians to Degrees2 : simulink_extras/Transformations/Radians to Degrees
  CurrPose : Outport
  wires:
  Bus Selector1/2 -> Mean/2(<X>1)  "<X>"
  Bus Selector1/1 -> Mean/1(<X>)  "<X>"
  Bus Selector1/5 -> Radians to Degrees1/1  "<psi>"
  Gain1/1 -> Mux1/4
  Bus Selector1/4 -> Mean1/2(<Y>1)  "<Y>"
  Mean1/1(Out1) -> Gain/1
  Gain/1 -> Mux1/2
  Gain3/1 -> Mux1/5
  Bus Selector1/8 -> Radians to Degrees2/1  "<theta>"
  Mean2/1(Out1) -> Gain1/1
  Bus Selector1/3 -> Mean1/1(<Y>)  "<Y>"
  Mean/1(Out1) -> Mux1/1
  Gain2/1 -> Mux1/3
  Radians to Degrees1/1 -> Gain2/1
  Bus Selector1/6 -> Mean2/1(<Z>)  "<Z>"
  Radians to Degrees2/1 -> Gain3/1
  Bus Selector1/7 -> Mean2/2(<Z>1)  "<Z>"
  Mux1/1 -> Math Function1/1
  Math Function1/1 -> CurrPose/1  "CurrPose"
  VehFdbk/1 -> Bus Selector1/1

== system TrajectoryFollowVehicleWith14DoF/Variant Subsystem/StanleyControl_vehicleDynamics/Vehicle Dynamics1/Vehicle Dynamics 3DOF/Calculate Norm ==
  Lateral Velocity : Inport
  Longitudinal Velocity : Inport  Port=2
  Add : Sum
  Math Function : Math  Operator=square
  Math Function1 : Math  Operator=square
  Sqrt : Sqrt
  Speed : Outport
  wires:
  Add/1 -> Sqrt/1
  Math Function1/1 -> Add/2
  Math Function/1 -> Add/1
  Sqrt/1 -> Speed/1
  Lateral Velocity/1 -> Math Function/1
  Longitudinal Velocity/1 -> Math Function1/1

== system TrajectoryFollowVehicleWith14DoF/Variant Subsystem/StanleyControl_vehicleDynamics/Vehicle Dynamics1/Vehicle Dynamics 3DOF/Delayed Steering System ==
  SteerCmd : Inport
  Add : Sum  Inputs=+-
  Delay : TransferFcn  Denominator=[0.1 0]
  CurrSteer : Outport  VectorParamsAs1DForOutWhenUnconnected=off
  wires:
  Add/1 -> Delay/1
  SteerCmd/1 -> Add/1
  Delay/1 -> CurrSteer/1, Add/2

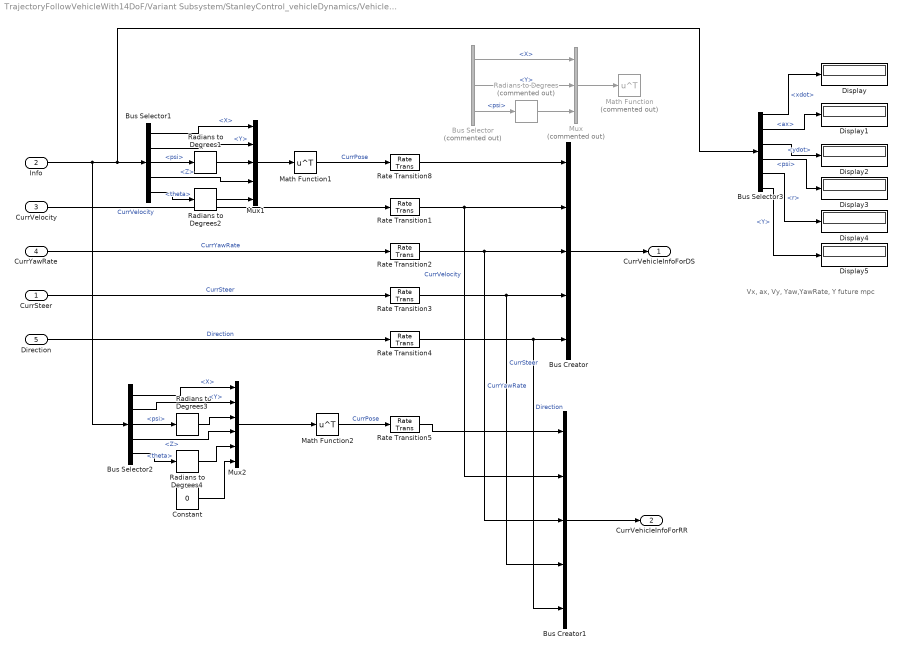
== system TrajectoryFollowVehicleWith14DoF/Variant Subsystem/StanleyControl_vehicleDynamics/Vehicle Dynamics1/Vehicle Dynamics 3DOF/Pack Current States ==
  note: Vx, ax, Vy, Yaw,YawRate, Y future mpc
  CurrSteer : Inport
  Info : Inport  Port=2
  CurrVelocity : Inport  Port=3
  CurrYawRate : Inport  Port=4
  Direction : Inport  Port=5
  Bus Creator : BusCreator  Inputs=5  OutDataTypeStr=Bus: BusVehicleInfo  NonVirtualBus=on
      settings: InheritFromInputs=off
  Bus Creator1 : BusCreator  Inputs=5  OutDataTypeStr=Bus: BusFullVehicleInfo  NonVirtualBus=on
      settings: InheritFromInputs=off
  Bus Selector : BusSelector  Commented=on  OutputSignals=InertFrm.RearAxl.Disp.X,InertFrm.RearAxl.Disp.Y,InertFrm.Cg.Ang.psi
  Bus Selector1 : BusSelector  OutputSignals=InertFrm.RearAxl.Disp.X,InertFrm.RearAxl.Disp.Y,InertFrm.Cg.Ang.psi,InertFrm.RearAxl.Disp.Z,InertFrm.Cg.Ang.theta
  Bus Selector2 : BusSelector  OutputSignals=InertFrm.Cg.Disp.X,InertFrm.Cg.Disp.Y,InertFrm.Cg.Ang.psi,InertFrm.Cg.Disp.Z,InertFrm.Cg.Ang.theta
  Bus Selector3 : BusSelector  OutputSignals=BdyFrm.Cg.Vel.xdot,BdyFrm.Cg.Acc.ax,BdyFrm.Cg.Vel.ydot,InertFrm.Cg.Ang.psi,BdyFrm.Cg.AngVel.r,InertFrm.Cg.Disp.Y
  Constant : Constant  Value=0
  Display{,1..5} (6 alike) : Display
  Math Function : Math  Commented=on  Operator=transpose  SignedPower=on
  Math Function1 : Math  Operator=transpose  SignedPower=on
  Math Function2 : Math  Operator=transpose  SignedPower=on
  Mux : Mux  Commented=on  Inputs=3
  Mux1 : Mux  Inputs=5
  Mux2 : Mux  Inputs=6
  Radians to Degrees : simulink_extras/Transformations/Radians to Degrees  Commented=on
  Radians to Degrees{1..4} (4 alike) : simulink_extras/Transformations/Radians to Degrees
  Rate Transition{1..5,8} (6 alike) : RateTransition  OutPortSampleTime=timeStep
  CurrVehicleInfoForDS : Outport  VectorParamsAs1DForOutWhenUnconnected=off
  CurrVehicleInfoForRR : Outport  Port=2  VectorParamsAs1DForOutWhenUnconnected=off
  wires:
  CurrVelocity/1 -> Rate Transition1/1  "CurrVelocity"
  CurrSteer/1 -> Rate Transition3/1  "CurrSteer"
  Math Function1/1 -> Rate Transition8/1  "CurrPose"
  CurrYawRate/1 -> Rate Transition2/1  "CurrYawRate"
  Direction/1 -> Rate Transition4/1  "Direction"
  Mux/1 -> Math Function/1
  Radians to Degrees/1 -> Mux/3
  Bus Selector/2 -> Mux/2  "<Y>"
  Bus Selector/1 -> Mux/1  "<X>"
  Bus Selector/3 -> Radians to Degrees/1  "<psi>"
  Bus Creator/1 -> CurrVehicleInfoForDS/1
  Rate Transition8/1 -> Bus Creator/1
  Bus Selector1/4 -> Mux1/4  "<Z>"
  Mux1/1 -> Math Function1/1
  Radians to Degrees1/1 -> Mux1/3
  Bus Selector1/2 -> Mux1/2  "<Y>"
  Bus Selector1/1 -> Mux1/1  "<X>"
  Bus Selector1/5 -> Radians to Degrees2/1  "<theta>"
  Radians to Degrees2/1 -> Mux1/5
  Bus Selector1/3 -> Radians to Degrees1/1  "<psi>"
  Rate Transition1/1 -> Bus Creator1/2, Bus Creator/2  "CurrVelocity"
  Radians to Degrees4/1 -> Mux2/5
  Bus Creator1/1 -> CurrVehicleInfoForRR/1
  Bus Selector2/4 -> Mux2/4  "<Z>"
  Bus Selector2/3 -> Radians to Degrees3/1  "<psi>"
  Rate Transition2/1 -> Bus Creator1/3, Bus Creator/3  "CurrYawRate"
  Radians to Degrees3/1 -> Mux2/3
  Bus Selector2/1 -> Mux2/1  "<X>"
  Rate Transition4/1 -> Bus Creator1/5, Bus Creator/5  "Direction"
  Mux2/1 -> Math Function2/1
  Math Function2/1 -> Rate Transition5/1  "CurrPose"
  Bus Selector2/2 -> Mux2/2  "<Y>"
  Rate Transition3/1 -> Bus Creator1/4, Bus Creator/4  "CurrSteer"
  Info/1 -> Bus Selector2/1, Bus Selector3/1, Bus Selector1/1
  Bus Selector2/5 -> Radians to Degrees4/1  "<theta>"
  Rate Transition5/1 -> Bus Creator1/1
  Constant/1 -> Mux2/6
  Bus Selector3/1 -> Display/1  "<xdot>"
  Bus Selector3/2 -> Display1/1  "<ax>"
  Bus Selector3/3 -> Display2/1  "<ydot>"
  Bus Selector3/4 -> Display3/1  "<psi>"
  Bus Selector3/5 -> Display4/1  "<r>"
  Bus Selector3/6 -> Display5/1  "<Y>"

== system TrajectoryFollowVehicleWith14DoF/Variant Subsystem/StanleyControl_vehicleDynamics/Vehicle Dynamics1/Vehicle Dynamics 3DOF/Simple Driveline & Brakes ==
  note: Trivial Driveline
  note: Trivial Powertrain
  note: Trivial Braking
  Accel : Inport
  Decel : Inport  Port=2
  Gear : Inport  Port=3
  xdot : Inport  Port=4
  Constant : Constant
  Gain : Gain  Gain=m
  Gain1 : Gain  Gain=0.8
  Gain2 : Gain  Gain=m
  Gain3 : Gain  Gain=0.5
  Lower level dynamics1 : TransferFcn  Denominator=[tau 1]
  Lower level dynamics2 : TransferFcn  Denominator=[tau2 1]
  Multiport Switch : MultiPortSwitch  DataPortOrder=Zero-based contiguous  zeroidx=on  SaturateOnIntegerOverflow=off  InputSameDT=off
  Neutral : Constant  Value=0
  Product : Product
  Saturation : Saturate  UpperLimit=1  LowerLimit=-1  ZeroCross=off
  Subtract1 : Sum  Inputs=+-
  Subtract2 : Sum
  Trigonometric Function : Trigonometry  Operator=tanh
  Unary Minus : UnaryMinus
  Front Force : Outport  VectorParamsAs1DForOutWhenUnconnected=off
  Rear Force : Outport  Port=2  VectorParamsAs1DForOutWhenUnconnected=off
  wires:
  Multiport Switch/1 -> Subtract1/1
  Accel/1 -> Gain/1
  xdot/1 -> Gain1/1
  Decel/1 -> Gain2/1
  Trigonometric Function/1 -> Product/2
  Gain1/1 -> Trigonometric Function/1
  Gain/1 -> Lower level dynamics1/1
  Gain2/1 -> Product/1
  Lower level dynamics2/1 -> Subtract1/2
  Product/1 -> Lower level dynamics2/1
  Gear/1 -> Saturation/1
  Constant/1 -> Subtract2/2
  Subtract2/1 -> Multiport Switch/1
  Neutral/1 -> Multiport Switch/3  "Neutral"
  Lower level dynamics1/1 -> Unary Minus/1, Multiport Switch/4  "Forward"
  Saturation/1 -> Subtract2/1
  Subtract1/1 -> Gain3/1  "Forward"
  Unary Minus/1 -> Multiport Switch/2  "Reverse"
  Gain3/1 -> Front Force/1, Rear Force/1
